simulink model "FinalProject"  (R2020a)
settings: Solver=VariableStepAuto  StartTime=0.0  StopTime=0.1  RelTol=1e-3
undefined symbols (not defined in the file): f1, f2, y
libraries: fl_lib x7, nesl_utility x7, eeGeneralControl x1, ee_lib x1
settings Model: OrderedModelArguments=off  Creator=colemanbeggs  LastModifiedBy=colemanbeggs

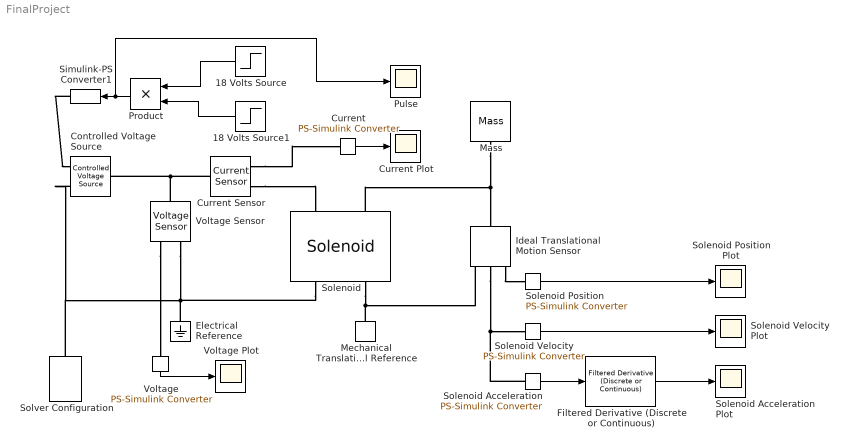
== system FinalProject ==
  18 Volts Source : Step  Time=y+0.01  Before=18  After=0  SampleTime=0
  18 Volts Source1 : Step  Time=y  SampleTime=0
  Controlled Voltage Source : fl_lib/Electrical/Electrical Sources/Controlled Voltage Source
  Current : nesl_utility/PS-Simulink Converter  PhysicalDomain=network_engine_domain  SubClassName=ps_output  LeftPortType=input  RightPortType=output  PseudoPeriodic=off  Frequencies=[]  Unit=inherit  AffineConversion=off
  Current Plot : Scope
  Current Sensor : fl_lib/Electrical/Electrical Sensors/Current Sensor
  Electrical Reference : fl_lib/Electrical/Electrical Elements/Electrical Reference
  Filtered Derivative (Discrete or Continuous) : eeGeneralControl/Filtered Derivative (Discrete or Continuous)  K=1  T=0.1  B=inf  A=-inf  minRatio=10  init_option=Inherited from block input  x0=0  Ts=-1
      settings: SourceProductBaseCode=PS
  Ideal Translational Motion Sensor : fl_lib/Mechanical/Mechanical Sensors/Ideal Translational Motion Sensor  offset=0 m
  Mass : fl_lib/Mechanical/Translational Elements/Mass  mass=30 g  v_specify=off  v_priority=High  v=0 m/s  v_nominal_specify=off  v_nominal_unit=m/s  v_nominal_value=1  f_specify=off  f_priority=None  f=0 N  f_nominal_specify=off  f_nominal_unit=N  f_nominal_value=1
  Mechanical Translational Reference : fl_lib/Mechanical/Translational Elements/Mechanical Translational Reference
  Product : Product
  Pulse : Scope
  Simulink-PS Converter1 : nesl_utility/Simulink-PS Converter  PhysicalDomain=network_engine_domain  SubClassName=ps_input  LeftPortType=input  RightPortType=output  PseudoPeriodic=off  Frequencies=[]  NoiseDistribution=none  NoiseParameters=[]  Unit=1  AffineConversion=off  FilteringAndDerivatives=provide  SimscapeFilterOrder=1  InputFilterTimeConstant=0.001  UdotUserProvided=0
  Solenoid : ee_lib/Electromechanical/Mechatronic Actuators/Solenoid  motionDirection=ee.enum.actuators.solenoidDirection.away  F12=[f1, f2] N  X12=[0.1, 0.5] in  K=0 N/m  Xzero=0 in  lam=0 N/(m/s)  Mass=9.01 g  Vdc=24 V  Imax=0.5 A  Xmax=0.5 in  K_endstop=545 N/m  D_endstop=1.0 N/(m/s)  i_specify=on  i_priority=High  i=0 mA  i_nominal_specify=off  i_nominal_unit=A  i_nominal_value=1  x_specify=on  x_priority=High  x=0 mm  x_nominal_specify=off  x_nominal_unit=mm  x_nominal_value=1  F_specify=off  F_priority=High  F=0 N  F_nominal_specify=off  F_nominal_unit=N  F_nominal_value=1  v_specify=off  v_priority=None  v=0 V  v_nominal_specify=off  v_nominal_unit=V  v_nominal_value=1  vel_specify=off  vel_priority=None  vel=0 m/s  vel_nominal_specify=off  vel_nominal_unit=m/s  vel_nominal_value=1  v_L_specify=off  v_L_priority=None  v_L=0 V  v_L_nominal_specify=off  v_L_nominal_unit=V  v_L_nominal_value=1  magnetic_force_specify=off  magnetic_force_priority=None  magnetic_force=0 N  magnetic_force_nominal_specify=off  magnetic_force_nominal_unit=N  magnetic_force_nominal_value=1  power_dissipated_specify=off  power_dissipated_priority=None  power_dissipated=0 W  power_dissipated_nominal_specify=off  power_dissipated_nominal_unit=W  power_dissipated_nominal_value=1  alpha=3.93e-3 1/K  Tmeas=25 degC  thermal_mass=100 J/K  temperature_specify=off  temperature_priority=High  temperature=25 degC  temperature_nominal_specify=off  temperature_nominal_unit=degC  temperature_nominal_value=1  Q_specify=off  Q_priority=None  Q=0 W  Q_nominal_specify=off  Q_nominal_unit=W  Q_nominal_value=1
      settings: SourceProductBaseCode=PS  InternalSimscapePortConfiguration="{\"Bottom\":[],\"Left\":[{\"id\":\"p\",\"label\":\"+\",\"type\":\"foundation.electrical.electrical\"},{\"id\":\"R\",\"label\":\"R\",\"type\":\"foundation.mechanical.translational.translational\"}],\"Right\":[{\"id\":\"n\",\"label\":\"-\",\"type\":\"foundation.electrical.electrical\"},{\"id\":\"C\",\"label\":\"C\",\"type\":\"foundation.mechanical.translational.translational\"}],\"Top\":[]}"
  Solenoid Acceleration : nesl_utility/PS-Simulink Converter  PhysicalDomain=network_engine_domain  SubClassName=ps_output  LeftPortType=input  RightPortType=output  PseudoPeriodic=off  Frequencies=[]  Unit=inherit  AffineConversion=off
  Solenoid Acceleration Plot : Scope
  Solenoid Position : nesl_utility/PS-Simulink Converter  PhysicalDomain=network_engine_domain  SubClassName=ps_output  LeftPortType=input  RightPortType=output  PseudoPeriodic=off  Frequencies=[]  Unit=inherit  AffineConversion=off
  Solenoid Position Plot : Scope
  Solenoid Velocity : nesl_utility/PS-Simulink Converter  PhysicalDomain=network_engine_domain  SubClassName=ps_output  LeftPortType=input  RightPortType=output  PseudoPeriodic=off  Frequencies=[]  Unit=inherit  AffineConversion=off
  Solenoid Velocity Plot : Scope
  Solver Configuration : nesl_utility/Solver Configuration  PhysicalDomain=network_engine_domain  SubClassName=solver  LeftPortType=input  RightPortType=generic  Tones=[]  Harmonics=[]  SimulateNoise=off  Profile=off  UseLocalSampling=off  EnableSwitchedLinearOptims=on  FrequencyDomain=off  UseCCode=off  RelTol=0.001  AbsTol=1e-06  MinStep=1e-09  ToWorkspace=off  RevertToSquareIcSolve=off  NumHomotopyIterations=100  PhasorMode=off  PhasorModeNumHarmonics=1  DoDC=off  ResidualTolerance=1e-09  UseLocalSolver=off  LocalSolverChoice=NE_BACKWARD_EULER_ADVANCER  LocalSolverSampleTime=0.001  DoFixedCost=off  MaxNonlinIter=3  MaxModeIter=2  LinearAlgebra=auto  EquationFormulation=NE_TIME_EF  DelaysMemoryBudget=1024  AutomaticFiltering=on  FilteringTimeConstant=0.001  PartitionStorageMethod=AS_NEEDED  PartitionMemoryBudget=1024  PartitionMethod=ROBUST
  Voltage : nesl_utility/PS-Simulink Converter  PhysicalDomain=network_engine_domain  SubClassName=ps_output  LeftPortType=input  RightPortType=output  PseudoPeriodic=off  Frequencies=[]  Unit=inherit  AffineConversion=off
  Voltage Plot : Scope
  Voltage Sensor : fl_lib/Electrical/Electrical Sensors/Voltage Sensor
  wires:
  Solenoid Velocity/1 -> Solenoid Velocity Plot/1
  Solenoid Position/1 -> Solenoid Position Plot/1
  Current/1 -> Current Plot/1
  Voltage/1 -> Voltage Plot/1
  Solenoid Acceleration/1 -> Filtered Derivative (Discrete or Continuous)/1
  Filtered Derivative (Discrete or Continuous)/1 -> Solenoid Acceleration Plot/1
  18 Volts Source/1 -> Product/1
  18 Volts Source1/1 -> Product/2
  Product/1 -> Pulse/1, Simulink-PS Converter1/1
  connections:
  Current Sensor/LConn1 -- Controlled Voltage Source/LConn1 -- Voltage Sensor/LConn1
  Solenoid/RConn1 -- Controlled Voltage Source/RConn2 -- Solver Configuration/RConn1 -- Electrical Reference/LConn1 -- Voltage Sensor/RConn2
  Current Sensor/RConn2 -- Solenoid/LConn1
  Solenoid/LConn2 -- Ideal Translational Motion Sensor/LConn1 -- Mass/LConn1
  Solenoid/RConn2 -- Mechanical Translational Reference/LConn1 -- Ideal Translational Motion Sensor/RConn1
  Current Sensor/RConn1 -- Current/LConn1
  Ideal Translational Motion Sensor/RConn3 -- Solenoid Position/LConn1
  Ideal Translational Motion Sensor/RConn2 -- Solenoid Acceleration/LConn1 -- Solenoid Velocity/LConn1
  Voltage Sensor/RConn1 -- Voltage/LConn1
  Simulink-PS Converter1/RConn1 -- Controlled Voltage Source/RConn1
